simulink model "RFCsvrTX_counter"  (Simulink 10.0)
settings: Solver=FixedStepDiscrete  StartTime=0.0  StopTime=inf  FixedStep=0.1  RelTol=1e-3
settings Model: Creator=fwornle  LastModifiedBy=bhisma  ExtModeTrigDuration=500
settings ConfigSet: Description=rtmc9s12target_R2009b
settings DataIOCC: LimitDataPoints=on  SignalLoggingSaveFormat=ModelDataLogs  SignalLoggingName=sigsOut
settings OptimizationCC: BooleanDataType=off  ExpressionDepthLimit=2147483647  InitFltsAndDblsToZero=on  LifeSpan=1  EfficientTunableParamExpr=on
settings DebuggingCC: SaveWithParameterizedLinksMsg=none  SignalResolutionControl=TryResolveAllWithWarning  MultiTaskDSMMsg=warning  MultiTaskCondExecSysMsg=none  FcnCallInpInsideContextMsg=warning  StateNameClashWarn=warning
settings HardwareCC: ProdBitPerInt=16  ProdBitPerPointer=16  ProdBitPerSizeT=16  ProdBitPerPtrDiffT=16  ProdEndianess=BigEndian  ProdWordSize=16  ProdHWDeviceType=Motorola HC12
settings SFSimCC: MATLABDynamicMemAlloc=off
settings RTWCC: SystemTargetFile=mc9s12.tlc  GenerateMakefile=off  TemplateMakefile=mc9s12.tmf
settings CodeAppCC: IgnoreCustomStorageClasses=off  CustomSymbolStrType=$N$R$M  InternalIdentifier=Classic
settings STFCustomTargetCC: TargetFcnLib=ansi_tfl_tmw.mat  ModelReferenceCompliant=off  IncludeMdlTerminateFcn=off  ERTCustomFileBanners=on  SupportNonInlinedSFcns=off  RemoveResetFunc=on  MATLABClassNameForMDSCustomization=Simulink.SoftwareTarget.ERTCustomization  CPPClassGenCompliant=on  SystemTargetFile=mc9s12.tlc
settings ERTTargetCC: TargetFcnLib=ansi_tfl_tmw.mat  MultiwordLength=2048  ModelReferenceCompliant=off  ParMdlRefBuildCompliant=off  CompOptLevelCompliant=off  ConcurrentExecutionCompliant=off  IncludeMdlTerminateFcn=off  CombineOutputUpdateFcns=off  SupportContinuousTime=on  ModelStepFunctionPrototypeControlCompliant=off  GRTInterface=on  UseToolchainInfoCompliant=off  ExtModeMexFile=ext_serial_mc9s12_comm  ExtModeMexArgs=1,2,115200  ERTCustomFileTemplate=mc9s12_file_process.tlc  ConvertIfToSwitch=off  SuppressUnreachableDefaultCases=off
settings CustomProperty: DataType=RTWOptions_EnumType_C__Users_fw__SVN_rtmc9s12-target_trunk_rtmc9s12_CW_R2009b_bin_mc9s12_1mc9s12_TargetBoard  Value=Dragon12Plus
settings EnumStrPairs: String=Dragon12
settings ConfigComp: CovExternalEMLEnable=off

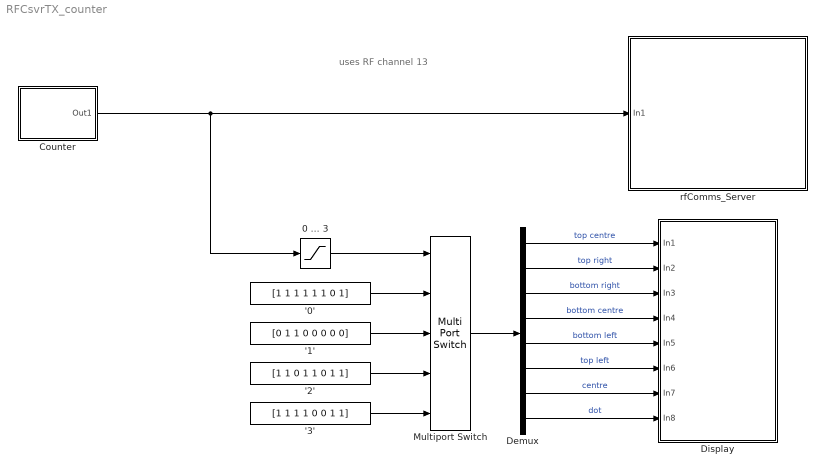
== system RFCsvrTX_counter ==
  note: uses RF channel 13
  '0' : Constant  Value=[1 1 1 1 1 1 0 1]  OutDataTypeStr=double
  '1' : Constant  Value=[0 1 1 0 0 0 0 0]  OutDataTypeStr=double
  '2' : Constant  Value=[1 1 0 1 1 0 1 1]  OutDataTypeStr=double
  '3' : Constant  Value=[1 1 1 1 0 0 1 1]  OutDataTypeStr=double
  0 ... 3 : Saturate  UpperLimit=3  LowerLimit=0
  Counter : Subsystem  mask{N=3, Ts=1}
      mask prompts: N "Final value"; Ts "Sample time"
  Demux : Demux  Outputs=8
  Display : Subsystem  Tag=mcTarget_digOut  mask{port=Port H, pin=0:7, sampletime=0.1, Von=0.5, Voff=0.5}
      mask prompts: port "Port (see hardware manuals for valid options)"; pin "Pin (see hardware manuals for valid options)"; sampletime "Sample time"; Von "On-threshold (Von)"; Voff "Off-threshold (Voff)"
      mask init:
      | [portstr, pinstr, pins] = mbc_digitaloutput(port, pin, sampletime, Von, Voff);
      mask Help: web('digOut_sfcn_9S12.html');
      mask TypeOptions port: Port A | Port B | Port H | Port J | Port M | Port P | Port S | Port T
      mask Display: fprintf('%s\nPins: %s', portstr, pinstr)
  Multiport Switch : MultiPortSwitch  DataPortOrder=Zero-based contiguous  Inputs=4  zeroidx=on  SaturateOnIntegerOverflow=on
  rfComms_Server : Subsystem  Tag=mcTarget_rfCommsSrv  mask{sampletime=0.1, RXTXmode=Transmission (TX), RFchannel=13, numClient=1, serverAddress=0xe7e7e7e7, clientAddress=0xc2c2c2c2, channel=0, buf_size=1, data_type=UINT8, format=on, outformat=on}
      mask prompts: sampletime "Sample time"; RXTXmode "Communication mode (TX, RX)"; RFchannel "RF channel number (0 - 127)"; numClient "Client to transmit to"; serverAddress "Server address (4 bytes, hexadecimal notation, e.g. 0xe7e7e7e7)"; clientAddress "Client address (4 bytes, hexadecimal notation, e.g.: 0xc2c2c2c2)"; channel "User channel number (0 - 9)"; buf_size "Number of elements to be sent/received"; data_type "Data Type"; format "Block sends/receives raw data"; outformat "Block output is 'double'"
      mask init:
      | [buf_sizestr, RXTXmodestr, RFchannelstr, clientstr, serverAddressstr, clientAddressstr, channelstr, data_type_str, sampletime_str] = mbc_rfComms_server(sampletime, RXTXmode, RFchannel, numClient, serverAddress, clientAddress, channel, buf_size, data_type, format, outformat);
      mask Help: web('rfComms_server.html');
      mask TypeOptions RXTXmode: Reception (RX) | Transmission (TX)
      mask TypeOptions numClient: 1 | 2 | 3 | 4 | 5
      mask TypeOptions data_type: SINGLE | INT8 | UINT8 | INT16 | UINT16 | INT32 | UINT32 | BOOLEAN
      mask Display: fprintf('RF mode: %s\nRF channel: %s\n%s\nServer address: %s\nClient address: %s\nUser channel: %s\nElements: %s\nData type: %s\n Sample rate: %s', RXTXmodestr, RFchannelstr, clientstr, serverAddressstr, clientAddressstr, channelstr, buf_sizestr, data_type_str, sampletime_str)
  wires:
  '0'/1 -> Multiport Switch/2
  '1'/1 -> Multiport Switch/3
  '2'/1 -> Multiport Switch/4
  Demux/1 -> Display/1(In1)  "top centre"
  Demux/2 -> Display/2(In2)  "top right"
  Demux/3 -> Display/3(In3)  "bottom right"
  Demux/4 -> Display/4(In4)  "bottom centre"
  Demux/5 -> Display/5(In5)  "bottom left"
  Demux/6 -> Display/6(In6)  "top left"
  Demux/7 -> Display/7(In7)  "centre"
  Demux/8 -> Display/8(In8)  "dot"
  Multiport Switch/1 -> Demux/1
  '3'/1 -> Multiport Switch/5
  0 ... 3/1 -> Multiport Switch/1
  Counter/1(Out1) -> 0 ... 3/1, rfComms_Server/1(In1)

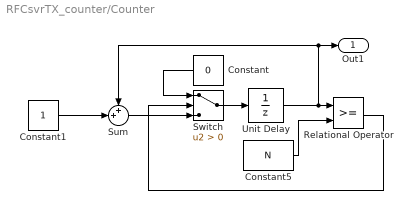
== system RFCsvrTX_counter/Counter ==
  Constant : Constant  Value=0
  Constant1 : Constant
  Constant5 : Constant  Value=N
  Relational Operator : RelationalOperator  OutDataTypeStr=uint(8)  RndMeth=Nearest
  Sum : Sum  Inputs=++|
  Switch : Switch  Criteria=u2 > Threshold
  Unit Delay : UnitDelay  SampleTime=Ts
  Out1 : Outport
  wires:
  Constant1/1 -> Sum/2
  Constant5/1 -> Relational Operator/2
  Constant/1 -> Switch/1
  Sum/1 -> Switch/3
  Unit Delay/1 -> Out1/1, Sum/1, Relational Operator/1
  Switch/1 -> Unit Delay/1
  Relational Operator/1 -> Switch/2

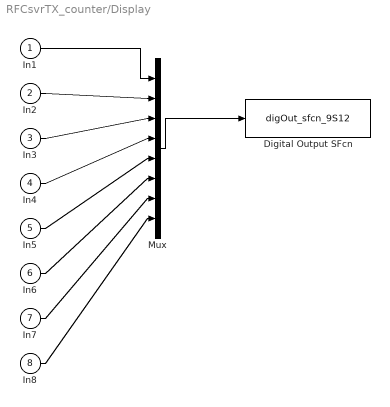
== system RFCsvrTX_counter/Display ==
  In1 : Inport
  In2 : Inport  Port=2
  In3 : Inport  Port=3
  In4 : Inport  Port=4
  In5 : Inport  Port=5
  In6 : Inport  Port=6
  In7 : Inport  Port=7
  In8 : Inport  Port=8
  Digital Output SFcn : S-Function  Tag=mcTarget_digOut  FunctionName=digOut_sfcn_9S12  Parameters=sampletime, port, pins, Von, Voff  SFunctionDeploymentMode=off  EnableBusSupport=off
  Mux : Mux  Inputs=8
  wires:
  Mux/1 -> Digital Output SFcn/1
  In1/1 -> Mux/1
  In2/1 -> Mux/2
  In3/1 -> Mux/3
  In4/1 -> Mux/4
  In5/1 -> Mux/5
  In6/1 -> Mux/6
  In7/1 -> Mux/7
  In8/1 -> Mux/8

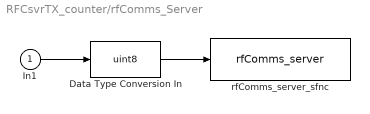
== system RFCsvrTX_counter/rfComms_Server ==
  In1 : Inport
  Data Type Conversion In : DataTypeConversion  OutDataTypeStr=uint8  SaturateOnIntegerOverflow=on  RndMeth=Zero
  rfComms_server_sfnc : S-Function  Tag=mcTarget_rfCommsSrv  FunctionName=rfComms_server  Parameters=sampletime, RXTXmode, channel, buf_size, data_type  SFunctionDeploymentMode=off  EnableBusSupport=off
  wires:
  Data Type Conversion In/1 -> rfComms_server_sfnc/1
  In1/1 -> Data Type Conversion In/1
